simulink model "simulink_w1"  (R2025a)
settings: Solver=VariableStepAuto  StartTime=0.0  StopTime=10.0  RelTol=1e-3
settings Model: Creator=luke_  LastModifiedBy=luke_

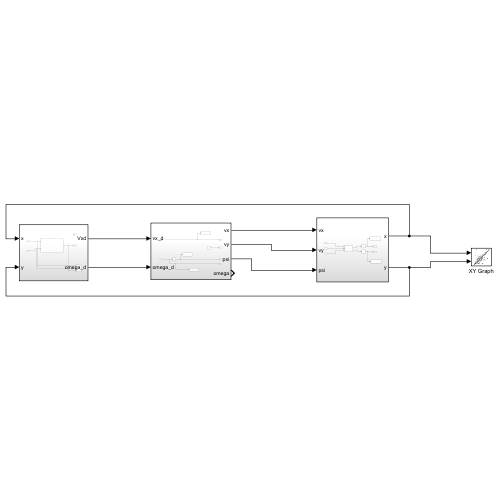
[thumbnail: Simulink's stored preview of the top-level diagram]
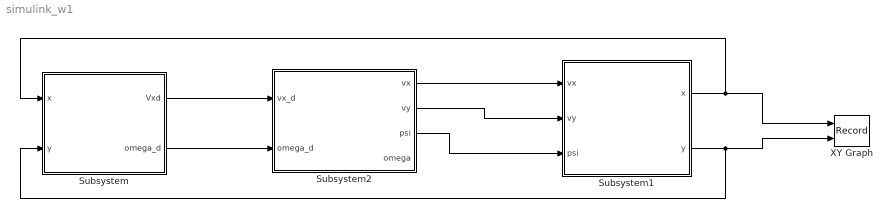
== system simulink_w1 ==
  Subsystem : Subsystem
  Subsystem1 : Subsystem
  Subsystem2 : Subsystem
  XY Graph : Record  NumPorts=2.0  FileSettingsInternal="{\"entries\":[{\"content\":{\"excelSettings\":{\"content\":{},\"type\":\"Streamout.ExcelSettings\"},\"parquetSettings\":{\"content\":{},\"type\":\"Streamout.ParquetSettings\"}},\"type\":\"Streamout.FileSettingStorage\",\"uuid\":\"\"}],\"packageUris\":[\"http:\\/\\/schema.mathworks.com\\/mf0\\/streamout_blocks\\/R2020a\"],\"version\":\"1.0\"}"  FrameSettings=[0, 0]  Layout=[1 1]  SignalsInternal="{\"entries\":[{\"content\":{\"signals\":[{\"content\":{\"blockPath\":[],\"dimensions\":[1],\"domain\":\"\",\"lineColor\":\"#a2142f\",\"plots\":[ 1 ],\"port\":1,\"sid\":[\"\"],\"signalID\":1,\"signalName\":\"Subsystem1:1\"},\"type\":\"RecordBlkView.Signal\",\"uuid\":\"\"},{\"content\":{\"blockPath\":[],\"dimensions\":[1],\"domain\":\"\",\"lineColor\":\"#139fff\",\"plots\":[ 1 ],\"port\":2,\"sid\":[\"\"],\"signalID\":2,\"signalName\":\"Subsystem1:2\"},\"type\":\"RecordBlkView.Signal\",\"uuid\":\"\"},{\"content\":{\"blockPath\":[],\"dimensions\":[1],\"domain\":\"\",\"lineColor\":\"#a2142f\",\"lineWidth\":2,\"port\":1,\"sid\":[\"\"],\"signalID\":3,\"signalName\":\"Integrator\"},\"type\":\"RecordBlkView.Signal\",\"uuid\":\"\"},{\"content\":{\"blockPath\":[],\"dimensions\":[1],\"domain\":\"\",\"lineColor\":\"#139fff\",\"lineWidth\":2,\"port\":1,\"sid\":[\"\"],\"signalID\":4,\"signalName\":\"Integrator1\"},\"type\":\"RecordBlkView.Signal\",\"uuid\":\"\"},{\"content\":{\"blockPath\":[],\"dimensions\":[1],\"domain\":\"\",\"lineColor\":\"#ff6929\",\"lineWidth\":2,\"port\":1,\"sid\":[\"\"],\"signalID\":5,\"signalName\":\"Integrator\"},\"type\":\"RecordBlkView.Signal\",\"uuid\":\"\"},{\"content\":{\"blockPath\":[],\"dimensions\":[1],\"domain\":\"\",\"lineColor\":\"#b746ff\",\"lineWidth\":2,\"port\":1,\"sid\":[\"\"],\"signalID\":6,\"signalName\":\"omega_d\"},\"type\":\"RecordBlkView.Signal\",\"uuid\":\"\"},{\"content\":{\"blockPath\":[],\"dimensions\":[1],\"domain\":\"\",\"lineColor\":\"#64d413\",\"lineWidth\":2,\"port\":1,\"sid\":[\"\"],\"signalID\":7,\"signalName\":\"vx_d\"},\"type\":\"RecordBlkView.Signal\",\"uuid\":\"\"}]},\"type\":\"RecordBlkView.InputSignals\",\"uuid\":\"\"}],\"packageUris\":[\"http:\\/\\/schema.mathworks.com\\/mf0\\/streamout_blocks\\/R2020a\"],\"version\":\"1.0\"}"  VisualizationBindings="{\"xyplotplugin\":{\"info\":[{\"series\":[{\"bindingParametersList\":[{\"parameter\":\"X-Axis\",\"signalID\":1,\"signalName\":\"Subsystem1:1\"},{\"parameter\":\"Y-Axis\",\"signalID\":2,\"signalName\":\"Subsystem1:2\"}],\"seriesID\":0}],\"subplotID\":1}]}}"  CompatibilityTag=XY
  wires:
  Subsystem/2(omega_d) -> Subsystem2/2(omega_d)
  Subsystem/1(Vxd) -> Subsystem2/1(vx_d)
  Subsystem2/1(vx) -> Subsystem1/1(vx)
  Subsystem2/2(vy) -> Subsystem1/2(vy)
  Subsystem2/3(psi) -> Subsystem1/3(psi)
  Subsystem1/1(x) -> Subsystem/1(x), XY Graph/1
  Subsystem1/2(y) -> Subsystem/2(y), XY Graph/2

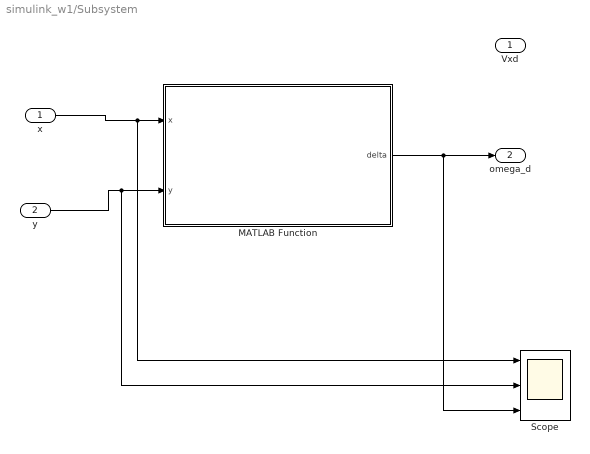
== system simulink_w1/Subsystem ==
  x : Inport
  y : Inport  Port=2
  MATLAB Function : MATLAB Function  TreatAsAtomicUnit=on
  Scope : Scope  NumInputPorts=3
  Vxd : Outport
  omega_d : Outport  Port=2
  wires:
  x/1 -> Scope/1, MATLAB Function/1(x)
  y/1 -> Scope/2, MATLAB Function/2(y)
  MATLAB Function/1(delta) -> Scope/3, omega_d/1

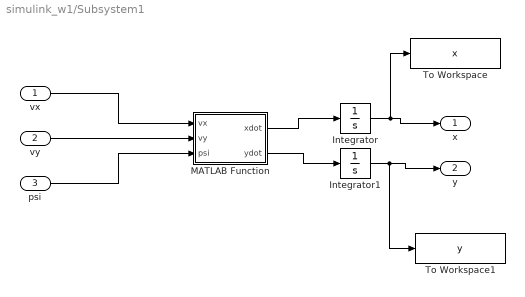
== system simulink_w1/Subsystem1 ==
  vx : Inport
  vy : Inport  Port=2
  psi : Inport  Port=3
  Integrator : Integrator
  Integrator1 : Integrator
  MATLAB Function : MATLAB Function  TreatAsAtomicUnit=on
  To Workspace : ToWorkspace  VariableName=x  SaveFormat=Timeseries  SampleTime=-1
  To Workspace1 : ToWorkspace  VariableName=y  SaveFormat=Timeseries  SampleTime=-1
  x : Outport
  y : Outport  Port=2
  wires:
  vx/1 -> MATLAB Function/1(vx)
  vy/1 -> MATLAB Function/2(vy)
  psi/1 -> MATLAB Function/3(psi)
  MATLAB Function/1(xdot) -> Integrator/1
  MATLAB Function/2(ydot) -> Integrator1/1
  Integrator/1 -> To Workspace/1, x/1
  Integrator1/1 -> To Workspace1/1, y/1

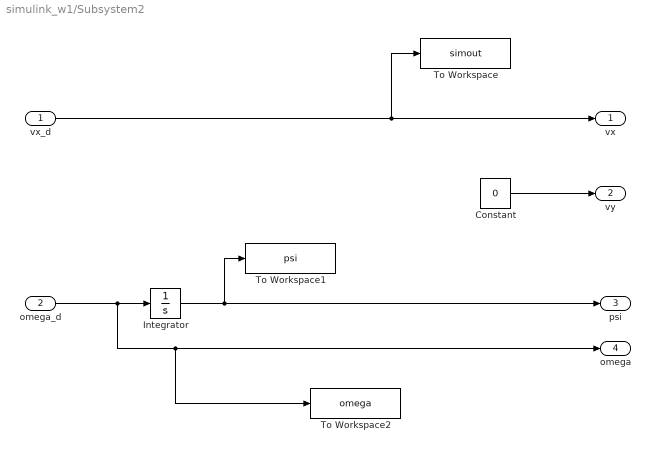
== system simulink_w1/Subsystem2 ==
  vx_d : Inport
  omega_d : Inport  Port=2
  Constant : Constant  Value=0
  Integrator : Integrator
  To Workspace : ToWorkspace  VariableName=simout  SaveFormat=Timeseries  SampleTime=-1
  To Workspace1 : ToWorkspace  VariableName=psi  SaveFormat=Timeseries  SampleTime=-1
  To Workspace2 : ToWorkspace  VariableName=omega  SaveFormat=Timeseries  SampleTime=-1
  vx : Outport
  vy : Outport  Port=2
  psi : Outport  Port=3
  omega : Outport  Port=4
  wires:
  omega_d/1 -> omega/1, To Workspace2/1, Integrator/1
  Integrator/1 -> To Workspace1/1, psi/1
  Constant/1 -> vy/1
  vx_d/1 -> To Workspace/1, vx/1

== matlab function simulink_w1/Subsystem/MATLAB Function ==
  data: x input; delta output; y input
function delta = simplestDriver(x,y)

if abs(y)<0.5
    delta = 0;
elseif abs(y-400) < 0.5
    delta = 0;
elseif x>900
    delta = 5;
else
    delta = -5;
end

== matlab function simulink_w1/Subsystem1/MATLAB Function ==
  data: vx input; xdot output; vy input; psi input; ydot output
function [xdot,ydot] = fcn(vx, vy, psi)
    temp = TF(psi)*[vx;vy];
    xdot = temp(1);
    ydot = temp(2);
end

function y = TF(psi)
    y = [cos(psi), -sin(psi);sin(psi),cos(psi)]
end
